simulink model "CartPendsys"  (R2022a)
settings: Solver=VariableStepAuto  StartTime=0.0  StopTime=10.0  RelTol=1e-3
values from neighbouring files (symbols this model uses):
  Kr_dis = lqr(sysC_dis.A,sysC_dis.B,Q,R)    [sim_pendcart.m]
  Mscale = [eye(4); zeros(2,4)]    [sim_pendcart.m]
  sysC = ss(A,BF,C,[0 0 0 0 0 Vn])    [sim_pendcart.m]
  x0 = [1.5 0 pi 0]    [sim_pendcart.m]
settings Model: Creator=samrudh.untgodpr  LastModifiedBy=samrudh.untgodpr
settings DebuggingCC: UnconnectedInputMsg=warning  UnconnectedOutputMsg=warning  UnconnectedLineMsg=warning
settings RTWCC: DLArmComputeVersion=19.05

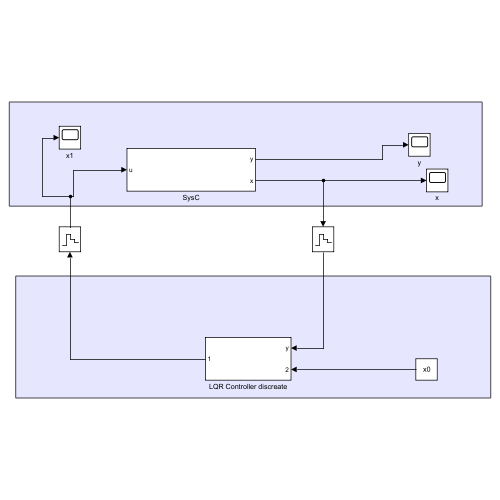
[thumbnail: Simulink's stored preview of the top-level diagram]
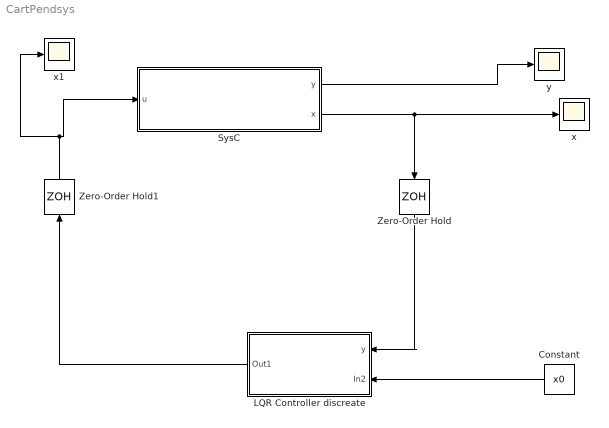
== system CartPendsys ==
  Constant : Constant  Value=x0
  LQR Controller discreate : Subsystem
  SysC : Subsystem
  Zero-Order Hold : ZeroOrderHold  SampleTime=-1
  Zero-Order Hold1 : ZeroOrderHold  SampleTime=0.01
  x : Scope
  x1 : Scope
  y : Scope
  wires:
  SysC/2(x) -> x/1, Zero-Order Hold/1
  LQR Controller discreate/1(Out1) -> Zero-Order Hold1/1
  Constant/1 -> LQR Controller discreate/2(In2)
  SysC/1(y) -> y/1
  Zero-Order Hold1/1 -> SysC/1(u), x1/1
  Zero-Order Hold/1 -> LQR Controller discreate/1(y)

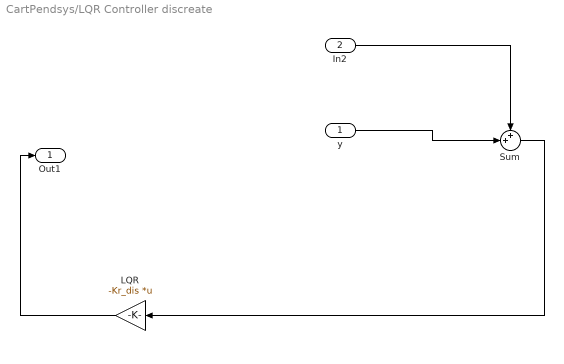
== system CartPendsys/LQR Controller discreate ==
  y : Inport
  In2 : Inport  Port=2
  LQR : Gain  Gain=-Kr_dis  Multiplication=Matrix(K*u) (u vector)
  Sum : Sum  Inputs=++|
  Out1 : Outport
  wires:
  LQR/1 -> Out1/1
  y/1 -> Sum/2
  In2/1 -> Sum/1
  Sum/1 -> LQR/1

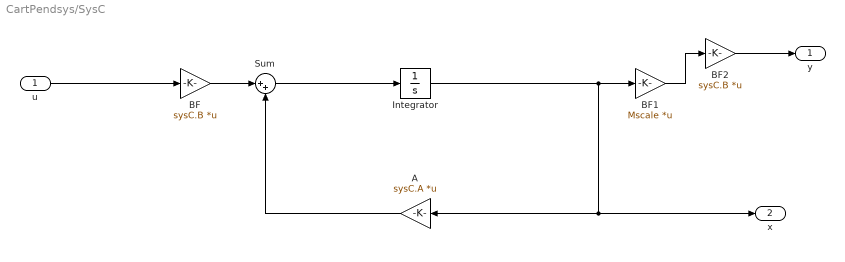
== system CartPendsys/SysC ==
  u : Inport  PortDimensions=6
  A : Gain  Gain=sysC.A  Multiplication=Matrix(K*u)
  BF : Gain  Gain=sysC.B  Multiplication=Matrix(K*u)
  BF1 : Gain  Gain=Mscale  Multiplication=Matrix(K*u)
  BF2 : Gain  Gain=sysC.B  Multiplication=Matrix(K*u) (u vector)
  Integrator : Integrator  InitialCondition=x0
  Sum : Sum  Inputs=|++
  y : Outport
  x : Outport  Port=2
  wires:
  Integrator/1 -> BF1/1, A/1, x/1
  A/1 -> Sum/2
  BF/1 -> Sum/1
  Sum/1 -> Integrator/1
  u/1 -> BF/1
  BF1/1 -> BF2/1
  BF2/1 -> y/1
